simulink model "washing_machine"  (R2024b)
settings: Solver=VariableStepAuto  StartTime=0.0  StopTime=inf  RelTol=1e-3
settings Model: Creator=Ajay1  LastModifiedBy=Ajay1

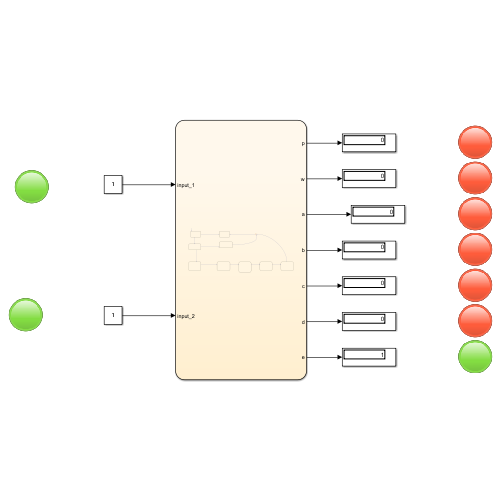
[thumbnail: Simulink's stored preview of the top-level diagram]
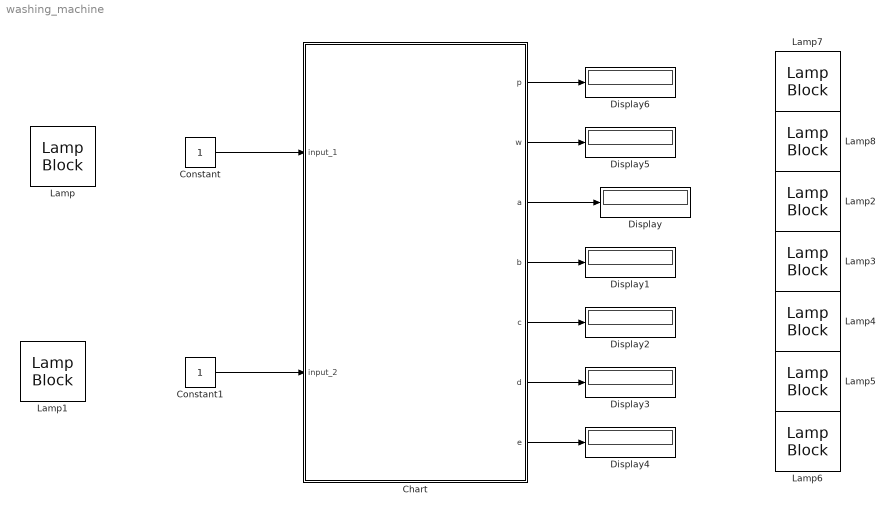
== system washing_machine ==
  Chart : Stateflow chart  TreatAsAtomicUnit=on
  Constant : Constant
  Constant1 : Constant
  Display{,1..6} (7 alike) : Display
  Lamp{,1..8} (9 alike) : LampBlock  LabelPosition=Hide
  wires:
  Constant/1 -> Chart/1(input_1)
  Constant1/1 -> Chart/2(input_2)
  Chart/3(a) -> Display/1
  Chart/4(b) -> Display1/1
  Chart/1(p) -> Display6/1
  Chart/2(w) -> Display5/1
  Chart/7(e) -> Display4/1
  Chart/6(d) -> Display3/1
  Chart/5(c) -> Display2/1

== stateflow chart washing_machine/Chart ==
  state powersupply_off
  state powersupply_on
    entry:
    p=1;
  state watersupply_off
  state watersupply_on
    entry:
    w=1
  state soaking
    entry:
    a=1;
    exit:
    a=0;
  state washing
    entry:
    b=1;
    exit:
    b=0;
  state rinsing
    entry:
    c=1;
    exit:
    c=0
    exit:
    w=0;
  state dryer
    entry:
    d=1;
    exit:
    d=0;
  state done
    entry:
    e=1;
    exit:
    p=0;
  (default) -> powersupply_on
  powersupply_on -> powersupply_off [order 1] : [input_1==0]
  (junction 33) -> powersupply_off
  done -> (junction 33)
  watersupply_off -> (junction 33)
  powersupply_on -> watersupply_on [order 2] : [input_1==1]
  watersupply_on -> watersupply_off [order 1] : [input_2==0]
  watersupply_on -> soaking [order 2] : [input_2==1]
  soaking -> washing : after(100,sec)
  washing -> rinsing : after(40,sec)
  rinsing -> dryer : after(60,sec)
  dryer -> done : after(70,sec)
  data: p output; w output; input_1 input; input_2 input; a output; b output; c output; d output; e output
